simulink model "demostration2"  (R2014b)
settings: Solver=ode45  StartTime=0.0  StopTime=60  RelTol=1e-3
settings Model: Creator=wangze  LastModifiedBy=wangze
settings DataIOCC: LimitDataPoints=off
settings OptimizationCC: UseDivisionForNetSlopeComputation=off  SimCompilerOptimization=off
settings DebuggingCC: FrameProcessingCompatibilityMsg=error  AllowSymbolicDim=off
settings RTWCC: RTWCompilerOptimization=off
settings ConfigComp: CovMetricSettings=dw  CovHtmlReporting=on  CovSaveCumulativeToWorkspaceVar=on  CovSaveSingleToWorkspaceVar=on  CovModelRefEnable=Off  CovExternalEMLEnable=off  CovSFcnEnable=off

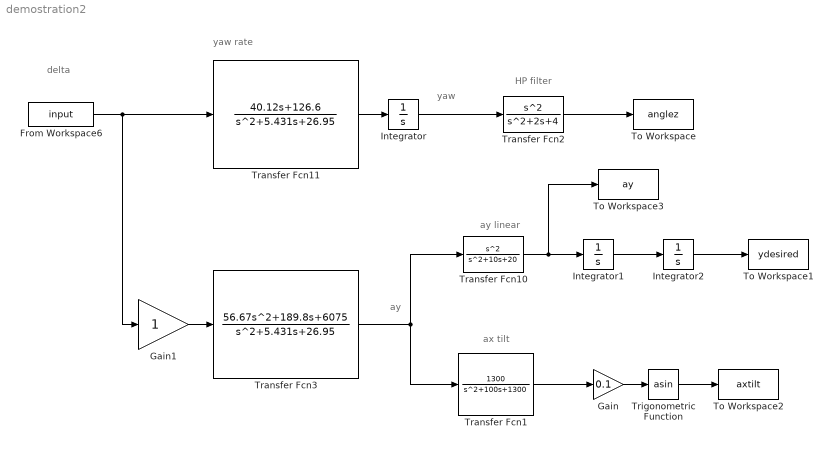
== system demostration2 ==
  note: ax tilt
  note: ay linear
  note: ay
  note: HP filter
  note: yaw
  note: yaw rate
  note: delta
  From Workspace6 : FromWorkspace  VariableName=input  SampleTime=0.05
  Gain : Gain  Gain=0.1
  Gain1 : Gain
  Integrator : Integrator
  Integrator1 : Integrator
  Integrator2 : Integrator
  To Workspace : ToWorkspace  VariableName=anglez  SampleTime=-1
  To Workspace1 : ToWorkspace  VariableName=ydesired  SampleTime=-1
  To Workspace2 : ToWorkspace  VariableName=axtilt  SampleTime=-1
  To Workspace3 : ToWorkspace  VariableName=ay  SampleTime=-1
  Transfer Fcn1 : TransferFcn  Numerator=[1300]  Denominator=[1 100 1300]
  Transfer Fcn10 : TransferFcn  Numerator=[1 0 0]  Denominator=[1 10 20]
  Transfer Fcn11 : TransferFcn  Numerator=[40.12 126.6]  Denominator=[1 5.431 26.95]
  Transfer Fcn2 : TransferFcn  Numerator=[1 0 0]  Denominator=[1 2 4]
  Transfer Fcn3 : TransferFcn  Numerator=[56.67 189.8 6075]  Denominator=[1 5.431 26.95]
  Trigonometric Function : Trigonometry  Operator=asin
  wires:
  From Workspace6/1 -> Gain1/1, Transfer Fcn11/1
  Transfer Fcn11/1 -> Integrator/1
  Integrator/1 -> Transfer Fcn2/1
  Transfer Fcn2/1 -> To Workspace/1
  Transfer Fcn3/1 -> Transfer Fcn1/1, Transfer Fcn10/1
  Transfer Fcn10/1 -> To Workspace3/1, Integrator1/1
  Integrator1/1 -> Integrator2/1
  Integrator2/1 -> To Workspace1/1
  Transfer Fcn1/1 -> Gain/1
  Gain/1 -> Trigonometric Function/1
  Gain1/1 -> Transfer Fcn3/1
  Trigonometric Function/1 -> To Workspace2/1
